simulink model "Unmodel_Dynamics_Ex21"  (R2023a)
settings: Solver=VariableStepAuto  StartTime=0.0  StopTime=100  RelTol=1e-3
undefined symbols (not defined in the file): gamma1, M_0, mi, q_0, sigma_0
settings Model: Creator=geokr  LastModifiedBy=geokr

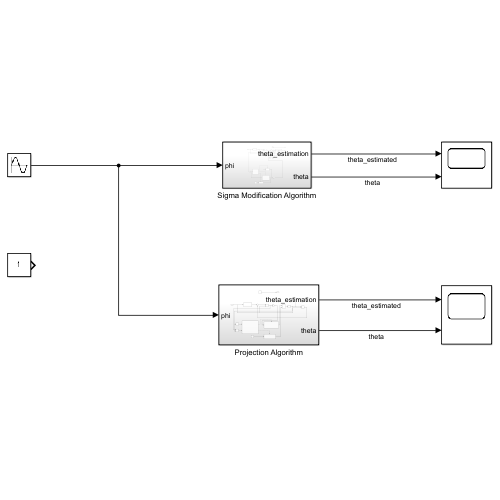
[thumbnail: Simulink's stored preview of the top-level diagram]
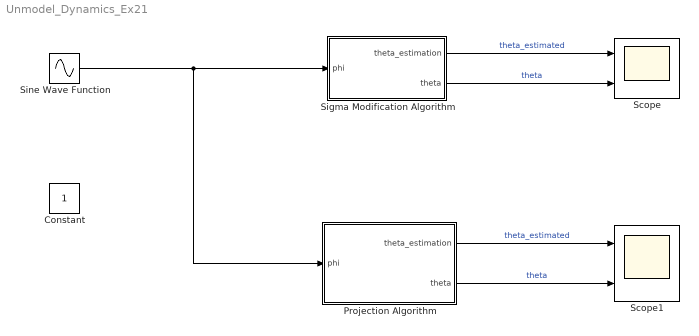
== system Unmodel_Dynamics_Ex21 ==
  Constant : Constant
  Projection Algorithm : Subsystem
  Scope : Scope  NumInputPorts=2
  Scope1 : Scope  NumInputPorts=2
  Sigma Modification Algorithm : Subsystem
  Sine Wave Function : Sin  SampleTime=0  VectorParams1D=off
  wires:
  Sigma Modification Algorithm/1(theta_estimation) -> Scope/1  "theta_estimated"
  Sigma Modification Algorithm/2(theta) -> Scope/2  "theta"
  Projection Algorithm/1(theta_estimation) -> Scope1/1  "theta_estimated"
  Projection Algorithm/2(theta) -> Scope1/2  "theta"
  Sine Wave Function/1 -> Sigma Modification Algorithm/1(phi), Projection Algorithm/1(phi)

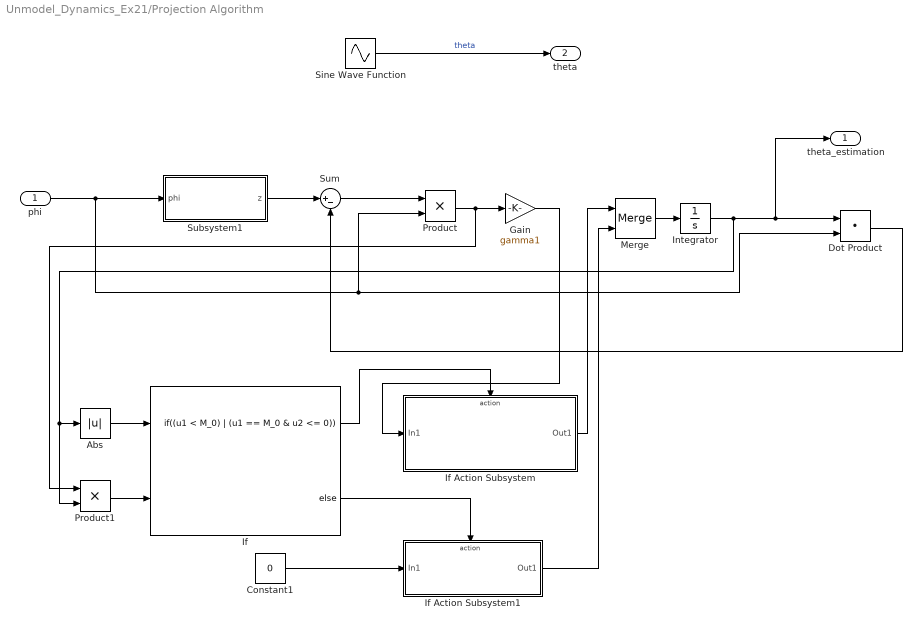
== system Unmodel_Dynamics_Ex21/Projection Algorithm ==
  phi : Inport
  Abs : Abs  SaturateOnIntegerOverflow=off
  Constant1 : Constant  Value=0
  Dot Product : DotProduct  OutDataTypeStr=Inherit: Inherit via internal rule
  Gain : Gain  Gain=gamma1
  If : If  NumInputs=2  IfExpression=(u1 < M_0) | (u1 == M_0 & u2 <= 0)
  If Action Subsystem : Subsystem  TreatAsAtomicUnit=on
  If Action Subsystem1 : Subsystem  TreatAsAtomicUnit=on
  Integrator : Integrator
  Merge : Merge
  Product : Product
  Product1 : Product
  Sine Wave Function : Sin  Bias=5  Frequency=0.1  SampleTime=0
  Subsystem1 : Subsystem
  Sum : Sum  Inputs=|+-
  theta_estimation : Outport
  theta : Outport  Port=2
  wires:
  Sine Wave Function/1 -> theta/1  "theta"
  phi/1 -> Dot Product/2, Product/2, Subsystem1/1(phi)
  Subsystem1/1(z) -> Sum/1
  Product/1 -> Product1/1, Gain/1
  Sum/1 -> Product/1
  Dot Product/1 -> Sum/2
  Integrator/1 -> Product1/2, Abs/1, theta_estimation/1, Dot Product/1
  Merge/1 -> Integrator/1
  Abs/1 -> If/1
  If/1 -> If Action Subsystem/Action
  If/2 -> If Action Subsystem1/Action
  If Action Subsystem/1(Out1) -> Merge/1
  If Action Subsystem1/1(Out1) -> Merge/2
  Gain/1 -> If Action Subsystem/1(In1)
  Constant1/1 -> If Action Subsystem1/1(In1)
  Product1/1 -> If/2

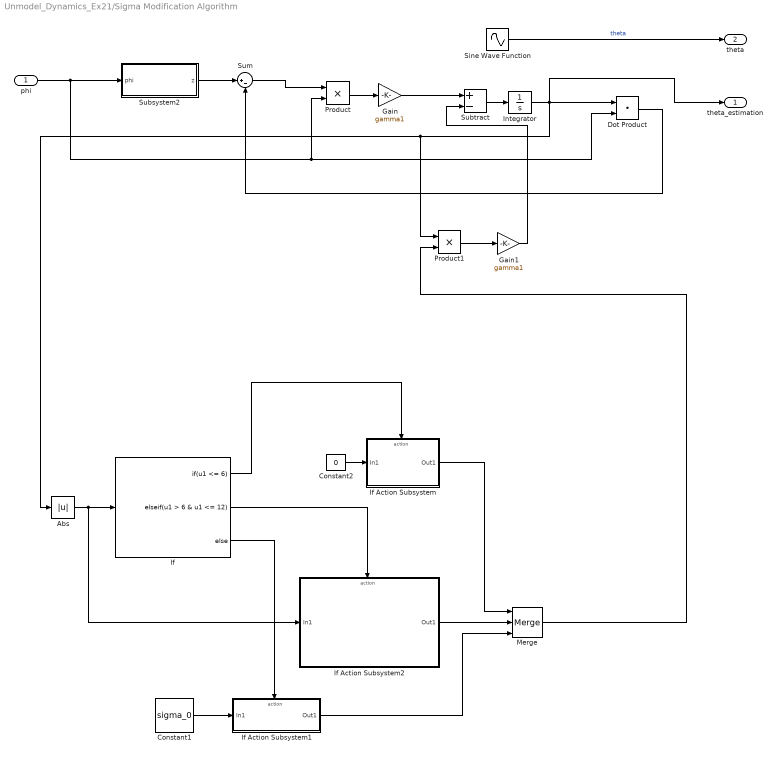
== system Unmodel_Dynamics_Ex21/Sigma Modification Algorithm ==
  phi : Inport
  Abs : Abs  SaturateOnIntegerOverflow=off
  Constant1 : Constant  Value=sigma_0
  Constant2 : Constant  Value=0
  Dot Product : DotProduct  OutDataTypeStr=Inherit: Inherit via internal rule
  Gain : Gain  Gain=gamma1
  Gain1 : Gain  Gain=gamma1
  If : If  IfExpression=u1 <= 6  ElseIfExpressions=u1 > 6 & u1 <= 12
  If Action Subsystem : Subsystem  TreatAsAtomicUnit=on
  If Action Subsystem1 : Subsystem  TreatAsAtomicUnit=on
  If Action Subsystem2 : Subsystem  TreatAsAtomicUnit=on
  Integrator : Integrator
  Merge : Merge  Inputs=3
  Product : Product
  Product1 : Product
  Sine Wave Function : Sin  Bias=5  Frequency=0.1  SampleTime=0
  Subsystem2 : Subsystem
  Subtract : Sum  Inputs=+-
  Sum : Sum  Inputs=|+-
  theta_estimation : Outport
  theta : Outport  Port=2
  wires:
  Sum/1 -> Product/1
  Product/1 -> Gain/1
  phi/1 -> Subsystem2/1(phi), Product/2, Dot Product/2
  Subsystem2/1(z) -> Sum/1
  Dot Product/1 -> Sum/2
  Gain/1 -> Subtract/1
  Subtract/1 -> Integrator/1
  Abs/1 -> If/1, If Action Subsystem2/1(In1)
  If Action Subsystem/1(Out1) -> Merge/1
  If Action Subsystem1/1(Out1) -> Merge/3
  If Action Subsystem2/1(Out1) -> Merge/2
  Merge/1 -> Product1/2
  Product1/1 -> Gain1/1
  Gain1/1 -> Subtract/2
  If/1 -> If Action Subsystem/Action
  If/2 -> If Action Subsystem2/Action
  If/3 -> If Action Subsystem1/Action
  Constant2/1 -> If Action Subsystem/1(In1)
  Constant1/1 -> If Action Subsystem1/1(In1)
  Sine Wave Function/1 -> theta/1  "theta"
  Integrator/1 -> Product1/1, Abs/1, theta_estimation/1, Dot Product/1

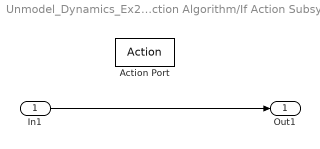
== system Unmodel_Dynamics_Ex21/Projection Algorithm/If Action Subsystem ==
  In1 : Inport
  Action Port : ActionPort  ActionPortLabel=if((u1 < M_0) | (u1 == M_0 & u2 <= 0))
  Out1 : Outport
  wires:
  In1/1 -> Out1/1

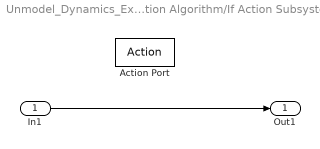
== system Unmodel_Dynamics_Ex21/Projection Algorithm/If Action Subsystem1 ==
  In1 : Inport
  Action Port : ActionPort  ActionPortLabel=else
  Out1 : Outport
  wires:
  In1/1 -> Out1/1

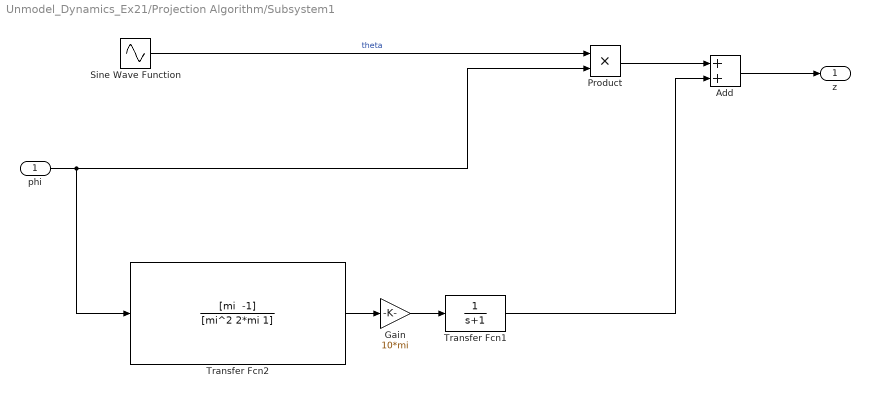
== system Unmodel_Dynamics_Ex21/Projection Algorithm/Subsystem1 ==
  phi : Inport
  Add : Sum
  Gain : Gain  Gain=10*mi
  Product : Product
  Sine Wave Function : Sin  Bias=5  Frequency=0.1  SampleTime=0
  Transfer Fcn1 : TransferFcn  Denominator=[1 1]
  Transfer Fcn2 : TransferFcn  Numerator="[mi  -1]"  Denominator=[mi^2 2*mi 1]
  z : Outport
  wires:
  Sine Wave Function/1 -> Product/1  "theta"
  phi/1 -> Product/2, Transfer Fcn2/1
  Transfer Fcn2/1 -> Gain/1
  Gain/1 -> Transfer Fcn1/1
  Transfer Fcn1/1 -> Add/2
  Product/1 -> Add/1
  Add/1 -> z/1

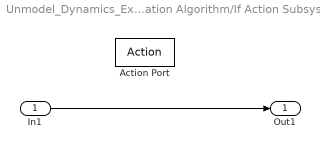
== system Unmodel_Dynamics_Ex21/Sigma Modification Algorithm/If Action Subsystem ==
  In1 : Inport
  Action Port : ActionPort  ActionPortLabel=if(u1 <= 6)
  Out1 : Outport
  wires:
  In1/1 -> Out1/1

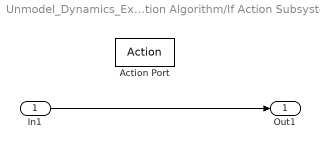
== system Unmodel_Dynamics_Ex21/Sigma Modification Algorithm/If Action Subsystem1 ==
  In1 : Inport
  Action Port : ActionPort  ActionPortLabel=else
  Out1 : Outport
  wires:
  In1/1 -> Out1/1

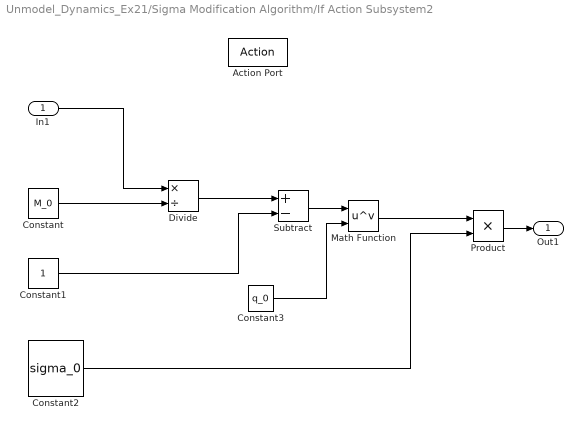
== system Unmodel_Dynamics_Ex21/Sigma Modification Algorithm/If Action Subsystem2 ==
  In1 : Inport
  Action Port : ActionPort  ActionPortLabel=elseif(u1 > 6 & u1 <= 12)
  Constant : Constant  Value=M_0
  Constant1 : Constant
  Constant2 : Constant  Value=sigma_0
  Constant3 : Constant  Value=q_0
  Divide : Product  Inputs=*/
  Math Function : Math  Operator=pow  OutputSignalType=real
  Product : Product
  Subtract : Sum  Inputs=+-
  Out1 : Outport
  wires:
  In1/1 -> Divide/1
  Constant/1 -> Divide/2
  Divide/1 -> Subtract/1
  Constant1/1 -> Subtract/2
  Constant2/1 -> Product/2
  Product/1 -> Out1/1
  Subtract/1 -> Math Function/1
  Math Function/1 -> Product/1
  Constant3/1 -> Math Function/2

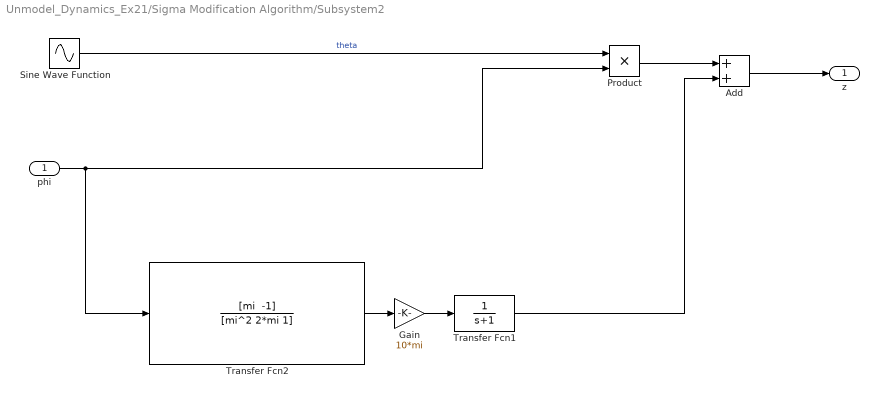
== system Unmodel_Dynamics_Ex21/Sigma Modification Algorithm/Subsystem2 ==
  phi : Inport
  Add : Sum
  Gain : Gain  Gain=10*mi
  Product : Product
  Sine Wave Function : Sin  Bias=5  Frequency=0.1  SampleTime=0
  Transfer Fcn1 : TransferFcn  Denominator=[1 1]
  Transfer Fcn2 : TransferFcn  Numerator="[mi  -1]"  Denominator=[mi^2 2*mi 1]
  z : Outport
  wires:
  Sine Wave Function/1 -> Product/1  "theta"
  phi/1 -> Product/2, Transfer Fcn2/1
  Transfer Fcn2/1 -> Gain/1
  Gain/1 -> Transfer Fcn1/1
  Transfer Fcn1/1 -> Add/2
  Product/1 -> Add/1
  Add/1 -> z/1
